simulink model "blockdemo"  (Simulink 6.3)
settings: Solver=VariableStepDiscrete  StartTime=0  StopTime=60  MaxStep=1  RelTol=1e-3
InitFcn:
  | %% DSPBuilder Start
  | alt_dspbuilder_update_model(bdroot)
  | %% DSPBuilder End
libraries: allblocks_alteradspbuilder2 x10
settings Model: Creator=mjervis  LastModifiedBy=delphick
settings OptimizationCC: BlockReduction=off  BooleanDataType=off  InlineInvariantSignals=on
settings DebuggingCC: SolverPrmCheckMsg=none
settings HardwareCC: TargetUnknown=on

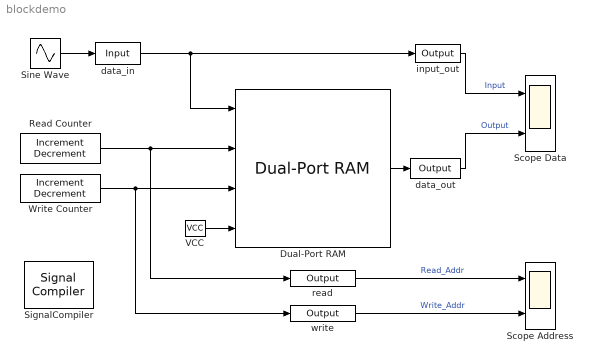
== system blockdemo ==
  Dual-Port RAM : allblocks_alteradspbuilder2/Dual-Port RAM  numwords=2^(7)  BusType=Inferred  bwl=8  bwr=0  memory_type=AUTO  ram_type=DualRAM  initialization=Blank  init_file=input.hex  init_array=[0:1:15]  register_outputs=off  use_ena=off  ClockPhase=1
  Read Counter : allblocks_alteradspbuilder2/Increment Decrement  BusType=Unsigned Integer  bwl=4  bwr=0  SpecifyClock=off  clr_value=0  direction=Increment  phase_selection=1  use_ena=off  use_sclr=off
  Scope Address : Scope  NumInputPorts=2
      settings: TimeRange=60  YMin=0~0  YMax=20~20  SampleInput=on  SampleTime=1
  Scope Data : Scope  NumInputPorts=2
      settings: TimeRange=60  YMin=-200~-200  YMax=200~200  SampleInput=on  SampleTime=1
  SignalCompiler : allblocks_alteradspbuilder2/Signal Compiler  DeviceFamily=Stratix IV  DeviceName=AUTO  EnableSignalTap=off  SignalTapDepth=128  UseBoardBlock=off  StpUseDefaultClock=on  StpClock=clock
  Sine Wave : Sin  SineType=Sample based  Amplitude=127  Frequency=0.25  Samples=25  SampleTime=1
  VCC : allblocks_alteradspbuilder2/VCC  SpecifyClock=off
  Write Counter : allblocks_alteradspbuilder2/Increment Decrement  BusType=Unsigned Integer  bwl=4  bwr=0  SpecifyClock=off  clr_value=0  direction=Increment  phase_selection=1  use_ena=off  use_sclr=off
  data_in : allblocks_alteradspbuilder2/Input  iofile=C:\workspace_clean\Documentation\DesignExamples\Tutorials\UnitBlocks\Storage\DualPortRAM\tb_blockdemo\blockdemo_data_in.salt  BusType=Signed Integer  bwl=8  bwr=8  SpecifyClock=off  PORTTYPE=Input
  data_out : allblocks_alteradspbuilder2/Output  iofile=C:\workspace_clean\Documentation\DesignExamples\Tutorials\UnitBlocks\Storage\DualPortRAM\tb_blockdemo\blockdemo_data_out.capture  BusType=Signed Integer  bwl=8  bwr=8  PORTTYPE=Output
  input_out : allblocks_alteradspbuilder2/Output  iofile=C:\workspace_clean\Documentation\DesignExamples\Tutorials\UnitBlocks\Storage\DualPortRAM\tb_blockdemo\blockdemo_input_out.capture  BusType=Signed Integer  bwl=8  bwr=8  PORTTYPE=Output
  read : allblocks_alteradspbuilder2/Output  iofile=C:\workspace_clean\Documentation\DesignExamples\Tutorials\UnitBlocks\Storage\DualPortRAM\tb_blockdemo\blockdemo_read.capture  BusType=Unsigned Integer  bwl=4  bwr=0  PORTTYPE=Output
  write : allblocks_alteradspbuilder2/Output  iofile=C:\workspace_clean\Documentation\DesignExamples\Tutorials\UnitBlocks\Storage\DualPortRAM\tb_blockdemo\blockdemo_write.capture  BusType=Unsigned Integer  bwl=4  bwr=0  PORTTYPE=Output
  wires:
  Sine Wave/1 -> data_in/1
  data_in/1 -> Dual-Port RAM/1, input_out/1
  Dual-Port RAM/1 -> data_out/1
  VCC/1 -> Dual-Port RAM/4
  Read Counter/1 -> Dual-Port RAM/2, read/1
  Write Counter/1 -> Dual-Port RAM/3, write/1
  data_out/1 -> Scope Data/2  "Output"
  read/1 -> Scope Address/1  "Read_Addr"
  write/1 -> Scope Address/2  "Write_Addr"
  input_out/1 -> Scope Data/1  "Input"
